simulink model "swpwm"  (Simulink 7.0)
settings: Solver=ode1  StartTime=0.0  StopTime=inf  FixedStep=0.0002  RelTol=1e-3
undefined symbols (not defined in the file): Model_626, Sensoray
libraries: rtwinlib x4, simulink x3, dsparch4 x1
settings Model: Creator=user  LastModifiedBy=user_2  SimulationMode=external  ExtModeTrigDuration=60000  BufferReuse=off
settings SolverCC: PositivePriorityOrder=on
settings DataIOCC: MaxDataPoints=60000
settings OptimizationCC: BooleanDataType=off  InlineInvariantSignals=on  OptimizeBlockIOStorage=off  BufferReuse=off  ExpressionFolding=off  LocalBlockOutputs=off
settings HardwareCC: TargetEndianess=LittleEndian  TargetHWDeviceType=MATLAB Host
settings RTWCC: SystemTargetFile=rtwin.tlc  TemplateMakefile=rtwin.tmf  Description=Real-Time Windows Target  ProcessScript=rtwin_make_rtw_hook
settings RTWinTargetCC: GenFloatMathFcnCalls=ANSI_C  ModelReferenceCompliant=off  CompOptLevelCompliant=off  PortableWordSizes=off  CCOptimize=on

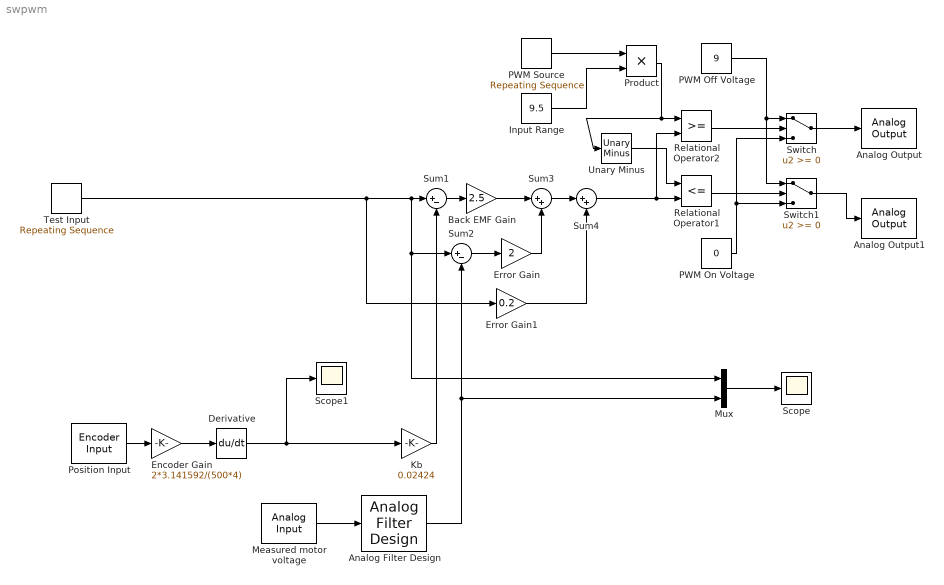
== system swpwm ==
  Analog Filter Design : dsparch4/Analog Filter Design  method=Butterworth  filttype=Lowpass  N=3  Wlo=100  Whi=80  Rp=2  Rs=40
  Analog Output : rtwinlib/Analog Output  SampleTime=-1  DrvName=Sensoray/Model_626  DrvAddress=4294967295  DrvOptions=zeros(1,0)  Channels=1  RangeMode=1  VoltRange=1  InitialValue=[]  FinalValue=[]
      settings: AttributesFormatString=Sensoray\nModel 626 [auto]
  Analog Output1 : rtwinlib/Analog Output  SampleTime=-1  DrvName=Sensoray/Model_626  DrvAddress=4294967295  DrvOptions=zeros(1,0)  Channels=2  RangeMode=1  VoltRange=1  InitialValue=[]  FinalValue=[]
      settings: AttributesFormatString=Sensoray\nModel 626 [auto]
  Back EMF Gain : Gain  Gain=2.5  ParameterDataType=sfix(16)  ParameterScaling=2^0  OutDataType=sfix(16)  OutScaling=2^0
  Derivative : Derivative
  Encoder Gain : Gain  Gain=2*3.141592/(500*4)  ParameterDataType=sfix(16)  ParameterScaling=2^0  OutDataType=sfix(16)  OutScaling=2^0
  Error Gain : Gain  Gain=2  ParameterDataType=sfix(16)  ParameterScaling=2^0  OutDataType=sfix(16)  OutScaling=2^0
  Error Gain1 : Gain  Gain=0.2  ParameterDataType=sfix(16)  ParameterScaling=2^0  OutDataType=sfix(16)  OutScaling=2^0
  Input Range : Constant  Value=9.5  OutDataType=sfix(16)  OutScaling=2^0
  Kb : Gain  Gain=0.02424  ParameterDataType=sfix(16)  ParameterScaling=2^0  OutDataType=sfix(16)  OutScaling=2^0
  Measured motor voltage : rtwinlib/Analog Input  SampleTime=-1  DrvName=Sensoray/Model_626  DrvAddress=4294967295  DrvOptions=zeros(1,0)  Channels=1  RangeMode=1  VoltRange=1  DataType=1
      settings: AttributesFormatString=Sensoray\nModel 626 [auto]
  Mux : Mux  Inputs=2
  PWM Off Voltage : Constant  Value=9  OutDataType=sfix(16)  OutScaling=2^0
  PWM On Voltage : Constant  Value=0  OutDataType=sfix(16)  OutScaling=2^0
  PWM Source : simulink/Sources/Repeating Sequence  SystemSampleTime=-1  rep_seq_t=[0 0.01]  rep_seq_y=[0 1]
  Position Input : rtwinlib/Encoder Input  SampleTime=-1  DrvName=Sensoray/Model_626  DrvAddress=4294967295  DrvOptions=zeros(1,0)  Channels=[4]  QuadMode=3  IndexPulse=2  InputFilter=Inf  DataType=1
      settings: AttributesFormatString=Sensoray\nModel 626 [auto]
  Product : Product  OutDataType=sfix(16)  OutScaling=2^0  RndMeth=Zero
  Relational Operator1 : RelationalOperator  Operator=<=  LogicOutDataTypeMode=boolean
  Relational Operator2 : RelationalOperator  LogicOutDataTypeMode=boolean
  Scope : Scope
      settings: TimeRange=60  YMin=-10  YMax=10  MaxDataPoints=60000
  Scope1 : Scope
      settings: TimeRange=60  YMin=-32.5  YMax=17.5  MaxDataPoints=60000
  Sum1 : Sum  Inputs=|+-  OutDataType=sfix(16)  OutScaling=2^0
  Sum2 : Sum  Inputs=|+-  OutDataType=sfix(16)  OutScaling=2^0
  Sum3 : Sum  Inputs=|++  OutDataType=sfix(16)  OutScaling=2^0
  Sum4 : Sum  Inputs=|++  OutDataType=sfix(16)  OutScaling=2^0
  Switch : Switch  OutDataType=sfix(16)  OutScaling=2^0
  Switch1 : Switch  OutDataType=sfix(16)  OutScaling=2^0
  Test Input : simulink/Sources/Repeating Sequence  SystemSampleTime=-1  rep_seq_t=[0 1 10 15 20 25 30 31 40 45 50 55 58 60]  rep_seq_y=[0 0 5 5 9.5 9.5 0 0 -5 -5 -9.5 -9.5 0 0]
  Unary Minus : simulink/Math Operations/Unary Minus  DoSatur=off
  wires:
  Relational Operator2/1 -> Switch/2
  Switch/1 -> Analog Output/1
  PWM Off Voltage/1 -> Switch/1, Switch1/1
  Relational Operator1/1 -> Switch1/2
  PWM On Voltage/1 -> Switch1/3, Switch/3
  Product/1 -> Relational Operator2/1, Unary Minus/1
  PWM Source/1 -> Product/1
  Input Range/1 -> Product/2
  Switch1/1 -> Analog Output1/1
  Measured motor voltage/1 -> Analog Filter Design/1
  Position Input/1 -> Encoder Gain/1
  Encoder Gain/1 -> Derivative/1
  Derivative/1 -> Kb/1, Scope1/1
  Test Input/1 -> Sum1/1, Sum2/1, Mux/1, Error Gain1/1
  Sum1/1 -> Back EMF Gain/1
  Kb/1 -> Sum1/2
  Sum2/1 -> Error Gain/1
  Back EMF Gain/1 -> Sum3/1
  Error Gain/1 -> Sum3/2
  Unary Minus/1 -> Relational Operator1/1
  Analog Filter Design/1 -> Sum2/2, Mux/2
  Mux/1 -> Scope/1
  Sum4/1 -> Relational Operator1/2, Relational Operator2/2
  Sum3/1 -> Sum4/1
  Error Gain1/1 -> Sum4/2
